simulink model "apf_pll"  (R2018a)
settings: Solver=ode1  StartTime=0  StopTime=40e-3  MaxStep=0.01  RelTol=0.1e-3
values from neighbouring files (symbols this model uses):
  R2 = 2    [mathematical_analysis.m]
undefined symbols (not defined in the file or in its folder): fs, pp
libraries: fl_lib x52, nesl_utility x17, powerlib x14, elec_lib x6, powerlib_extras x4, simulink x4, powerlib_meascontrol x1
settings Model: Creator=rodrigo  LastModifiedBy=LASAGNA
settings SolverCC: MaxConsecutiveZCs=10000  ShapePreserveControl=EnableAll  ZeroCrossControl=EnableAll
settings DataIOCC: SaveFormat=Array  SignalLoggingSaveFormat=ModelDataLogs  SaveOutput=off  SaveTime=off
settings OptimizationCC: BooleanDataType=off  ExpressionDepthLimit=2147483647  InitFltsAndDblsToZero=on  LifeSpan=inf
settings DebuggingCC: SaveWithParameterizedLinksMsg=none  UnderspecifiedInitializationDetection=Classic  MergeDetectMultiDrivingBlocksExec=none  SignalResolutionControl=TryResolveAllWithWarning  MultiTaskDSMMsg=warning  MultiTaskCondExecSysMsg=none  FcnCallInpInsideContextMsg=warning  StateNameClashWarn=warning  SFUnexpectedBacktrackingDiag=warning  SFNoUnconditionalDefaultTransitionDiag=warning  SFExecutionAtInitializationDiag=none
settings HardwareCC: ProdBitPerPointer=32  ProdBitPerSizeT=32  ProdBitPerPtrDiffT=32  ProdLargestAtomicFloat=None  ProdIntDivRoundTo=Undefined  ProdEndianess=Unspecified  ProdWordSize=32  ProdHWDeviceType=32-bit Generic  TargetBitPerPointer=64  TargetBitPerSizeT=64  TargetBitPerPtrDiffT=64  TargetLongLongMode=on  TargetIntDivRoundTo=Zero  TargetEndianess=LittleEndian  TargetWordSize=64  TargetHWDeviceType=MATLAB Host  ProdEqTarget=off
settings ModelReferenceCC: PropagateSignalLabelsOutOfModel=off
settings CodeAppCC: StateflowObjectComments=on
settings GRTTargetCC: TargetFcnLib=ansi_tfl_tmw.mat  TargetLangStandard=C89/C90 (ANSI)  CombineOutputUpdateFcns=off  GRTInterface=on
settings ConfigComp: CovMetricSettings=dw  CovHtmlReporting=on  CovSaveCumulativeToWorkspaceVar=on  CovSaveSingleToWorkspaceVar=on  CovExternalEMLEnable=off
settings SimscapeCC: SimscapeNormalizeSystem=off

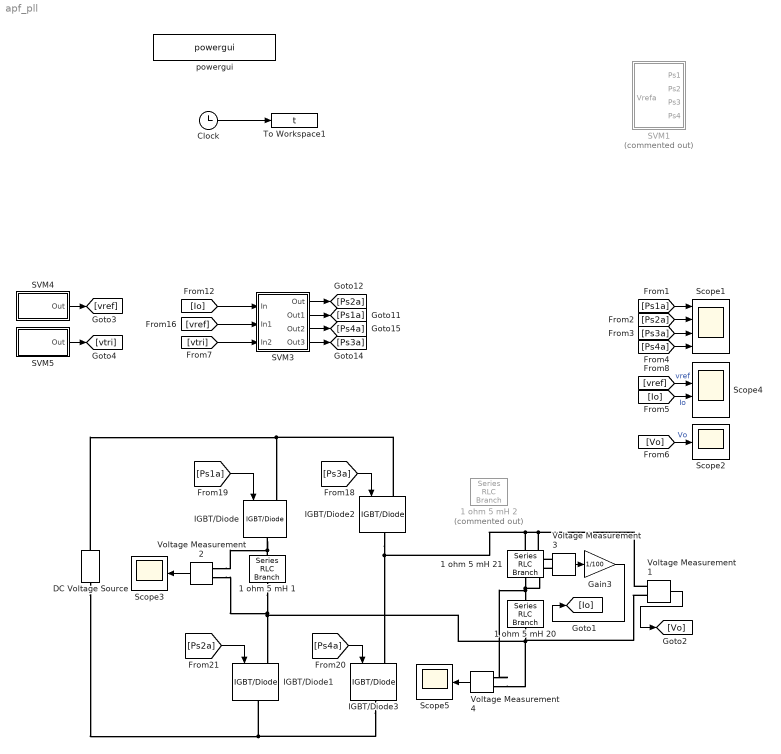
== system apf_pll ==
  1 ohm 5 mH 1 : powerlib/Elements/Series RLC Branch  LConnTagsString=__new0  RConnTagsString=__new0  BranchType=R  Resistance=1  Inductance=5e-03  SetiL0=off  InitialCurrent=0  Capacitance=0.001  Setx0=off  InitialVoltage=0  Measurements=None
  1 ohm 5 mH 2 : powerlib/Elements/Series RLC Branch  Commented=on  LConnTagsString=__new0  RConnTagsString=__new0  BranchType=R  Resistance=R2  Inductance=5e-03  SetiL0=off  InitialCurrent=0  Capacitance=0.001  Setx0=off  InitialVoltage=0  Measurements=None
  1 ohm 5 mH 20 : powerlib/Elements/Series RLC Branch  LConnTagsString=__new0  RConnTagsString=__new0  BranchType=L  Resistance=100  Inductance=0.256  SetiL0=off  InitialCurrent=10  Capacitance=60u  Setx0=off  InitialVoltage=0  Measurements=None
  1 ohm 5 mH 21 : powerlib/Elements/Series RLC Branch  LConnTagsString=__new0  RConnTagsString=__new0  BranchType=R  Resistance=100  Inductance=5e-03  SetiL0=off  InitialCurrent=0  Capacitance=0.001  Setx0=off  InitialVoltage=0  Measurements=None
  Clock : Clock
  DC Voltage Source : powerlib/Electrical Sources/DC Voltage Source  Amplitude=60  Measurements=None
  Gain3 : Gain  Gain=1/100
  IGBT/Diode{,1..3} (4 alike) : powerlib/Power Electronics/IGBT//Diode  Ron=1e-3  Rs=1e5  Cs=inf  Measurements=off
  SVM1 : Subsystem  Commented=on
  SVM3 : Subsystem
  SVM4 : Subsystem
  SVM5 : Subsystem
  Scope1 : Scope  NumInputPorts=4
  Scope2 : Scope
  Scope3 : Scope
  Scope4 : Scope  NumInputPorts=4
  Scope5 : Scope
  To Workspace1 : ToWorkspace  VariableName=t
      settings: MaxDataPoints=2000000
  Voltage Measurement{1..4} (4 alike) : powerlib/Measurements/Voltage Measurement  PhasorSimulation=off  OutputType=Complex  PSBequivalent=0
  powergui : powerlib/powergui  Priority=1  SimulationMode=Discrete  SampleTime=1/150e4  frequency=60  Iterations=50  frequencyindice=0  Pbase=100e6  ErrMax=1e-4  UnitsV=kV  UnitsW=MW  buscounter=0  FunctionMessages=off  echomessages=off  EnableUseOfTLC=off  CurrentSourceSwitches=off  DisableSnubberDevices=off  DisableRonSwitches=off  DisableVfSwitches=off  DisplayEquations=off  SolverType=Tustin/Backward Euler (TBE)  Interpol=off  ExternalGateDelay=off  methode=off  Ts=0  x0status=blocks  SPID=on  SwTol=0  HookPort=off  RestoreLinks=warning  ResistiveCurrentMeasurement=off  Frange=[0:2:500]  Ylog=off  Xlog=on  ShowGrid=off  save=off  variable=ZData  structure=ISA  ZoomFFT=off  StartTime=0.1  cycles=3  DisplayStyle=1  fundamental=60  FreqAxis=off  MaxFrequency=1000  frequencyindicesteady=1  RmsSteady=1  display=off
  wires:
  Clock/1 -> To Workspace1/1
  [Ps3a] -> IGBT/Diode2/1
  [Ps1a] -> IGBT/Diode/1
  [Ps4a] -> IGBT/Diode3/1
  [Ps2a] -> IGBT/Diode1/1
  [Ps1a] -> Scope1/1
  [Ps2a] -> Scope1/2
  [Ps3a] -> Scope1/3
  [Ps4a] -> Scope1/4
  Voltage Measurement3/1 -> Gain3/1
  Gain3/1 -> [Io]
  Voltage Measurement1/1 -> [Vo]
  SVM4/1(Out) -> [vref]
  [Vo] -> Scope2/1  "Vo"
  [vref] -> Scope4/2  "vref"
  [Io] -> Scope4/3  "Io"
  ? -> Scope4/1  "err"
  [Io] -> SVM3/1(In)
  ? -> Scope4/4  "IoxKh"
  [vref] -> SVM3/2(In1)
  SVM5/1(Out) -> [vtri]
  [vtri] -> SVM3/3(In2)
  SVM3/4(Out3) -> [Ps3a]
  SVM3/3(Out2) -> [Ps4a]
  SVM3/1(Out) -> [Ps2a]
  SVM3/2(Out1) -> [Ps1a]
  Voltage Measurement2/1 -> Scope3/1
  Voltage Measurement4/1 -> Scope5/1
  connections:
  Voltage Measurement1/LConn2 -- Voltage Measurement4/LConn2 -- 1 ohm 5 mH 20/LConn1 -- 1 ohm 5 mH 1/LConn1 -- Voltage Measurement2/LConn2 -- IGBT/Diode1/LConn1
  IGBT/Diode3/RConn1 -- IGBT/Diode1/RConn1 -- DC Voltage Source/LConn1
  IGBT/Diode2/LConn1 -- IGBT/Diode/LConn1 -- DC Voltage Source/RConn1
  1 ohm 5 mH 21/LConn1 -- 1 ohm 5 mH 20/RConn1 -- Voltage Measurement3/LConn2 -- Voltage Measurement4/LConn1
  1 ohm 5 mH 21/RConn1 -- Voltage Measurement1/LConn1 -- Voltage Measurement3/LConn1 -- IGBT/Diode2/RConn1 -- IGBT/Diode3/LConn1
  1 ohm 5 mH 1/RConn1 -- Voltage Measurement2/LConn1 -- IGBT/Diode/RConn1

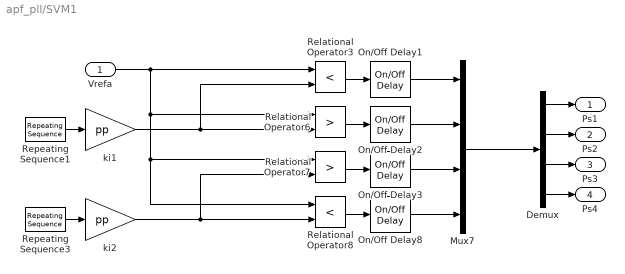
== system apf_pll/SVM1 ==
  Vrefa : Inport
  Demux : Demux
  Mux7 : Mux
  On/Off Delay{1..3,8} (4 alike) : powerlib_extras/Control  Blocks/On//Off Delay  type_delay=On delay  delay=tm  ic=0
  Relational Operator3 : RelationalOperator  Operator=<  OutDataTypeStr=boolean  RndMeth=Nearest
  Relational Operator6 : RelationalOperator  Operator=>  OutDataTypeStr=boolean  RndMeth=Nearest
  Relational Operator7 : RelationalOperator  Operator=>  OutDataTypeStr=boolean  RndMeth=Nearest
  Relational Operator8 : RelationalOperator  Operator=<  OutDataTypeStr=boolean  RndMeth=Nearest
  Repeating Sequence1 : simulink/Sources/Repeating Sequence  rep_seq_t=[0 1/(2*fs) 1/fs]  rep_seq_y=[0 1 0]
  Repeating Sequence3 : simulink/Sources/Repeating Sequence  rep_seq_t=[0 1/(2*fs) 1/fs]  rep_seq_y=[1 0 1]
  ki1 : Gain  Gain=pp  SaturateOnIntegerOverflow=on  OutDataTypeStr=Inherit: Same as input  ParamDataTypeStr=Inherit: Same as input
  ki2 : Gain  Gain=pp  SaturateOnIntegerOverflow=on  OutDataTypeStr=Inherit: Same as input  ParamDataTypeStr=Inherit: Same as input
  Ps1 : Outport
  Ps2 : Outport  Port=2
  Ps3 : Outport  Port=3
  Ps4 : Outport  Port=4
  wires:
  Vrefa/1 -> Relational Operator3/1, Relational Operator7/1, Relational Operator8/1, Relational Operator6/1
  Repeating Sequence1/1 -> ki1/1
  ki1/1 -> Relational Operator3/2, Relational Operator6/2
  ki2/1 -> Relational Operator8/2, Relational Operator7/2
  Repeating Sequence3/1 -> ki2/1
  Relational Operator3/1 -> On/Off Delay1/1
  Relational Operator6/1 -> On/Off Delay2/1
  Relational Operator7/1 -> On/Off Delay3/1
  Relational Operator8/1 -> On/Off Delay8/1
  On/Off Delay2/1 -> Mux7/2
  On/Off Delay1/1 -> Mux7/1
  On/Off Delay3/1 -> Mux7/3
  On/Off Delay8/1 -> Mux7/4
  Demux/1 -> Ps1/1
  Demux/2 -> Ps2/1
  Demux/3 -> Ps3/1
  Demux/4 -> Ps4/1
  Mux7/1 -> Demux/1

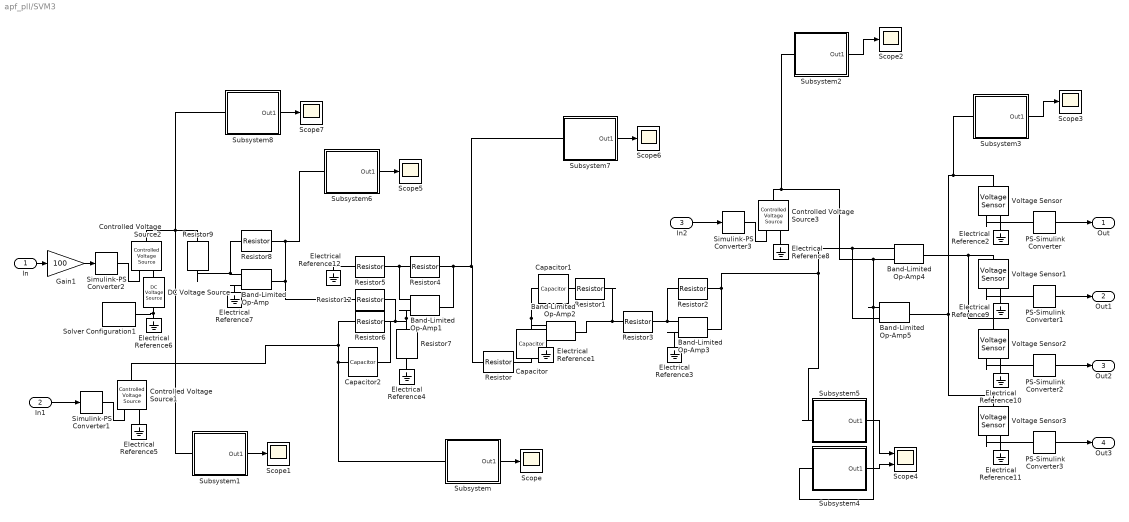
== system apf_pll/SVM3 ==
  In : Inport
  In1 : Inport  Port=2
  In2 : Inport  Port=3
  Band-Limited Op-Amp{,1..3} (4 alike) : elec_lib/Integrated Circuits/Band-Limited Op-Amp  A=25000  Rin=1e12 Ohm  Rout=50 Ohm  Vmin=-15 V  Vmax=15 V  Vdotmax=1e5 V/s  f=3 GHz  V0=0 V
      settings: SourceProductName=Simscape Electronics  SourceProductBaseCode=SN
  Band-Limited Op-Amp4 : elec_lib/Integrated Circuits/Band-Limited Op-Amp  A=25000  Rin=1e12 Ohm  Rout=50 Ohm  Vmin=0 V  Vmax=5 V  Vdotmax=1e5 V/s  f=3 GHz  V0=0 V
      settings: SourceProductName=Simscape Electronics  SourceProductBaseCode=SN
  Band-Limited Op-Amp5 : elec_lib/Integrated Circuits/Band-Limited Op-Amp  A=25000  Rin=1e12 Ohm  Rout=50 Ohm  Vmin=0 V  Vmax=5 V  Vdotmax=1e5 V/s  f=3 GHz  V0=0 V
      settings: SourceProductName=Simscape Electronics  SourceProductBaseCode=SN
  Capacitor : fl_lib/Electrical/Electrical Elements/Capacitor  c=100 nF  r=1e-6 Ohm  g=1e-9 1/Ohm  i_specify=off  i_priority=None  i=0 A  i_nominal_specify=off  i_nominal_unit=A  i_nominal_value=1  v_specify=off  v_priority=None  v=0 V  v_nominal_specify=off  v_nominal_unit=V  v_nominal_value=1  vc_specify=off  vc_priority=High  vc=0 V  vc_nominal_specify=off  vc_nominal_unit=V  vc_nominal_value=1
  Capacitor1 : fl_lib/Electrical/Electrical Elements/Capacitor  c=100 nF  r=1e-6 Ohm  g=1e-9 1/Ohm  i_specify=off  i_priority=None  i=0 A  i_nominal_specify=off  i_nominal_unit=A  i_nominal_value=1  v_specify=off  v_priority=None  v=0 V  v_nominal_specify=off  v_nominal_unit=V  v_nominal_value=1  vc_specify=off  vc_priority=High  vc=0 V  vc_nominal_specify=off  vc_nominal_unit=V  vc_nominal_value=1
  Capacitor2 : fl_lib/Electrical/Electrical Elements/Capacitor  c=100 nF  r=1e-6 Ohm  g=1e-9 1/Ohm  i_specify=off  i_priority=None  i=0 A  i_nominal_specify=off  i_nominal_unit=A  i_nominal_value=1  v_specify=off  v_priority=None  v=0 V  v_nominal_specify=off  v_nominal_unit=V  v_nominal_value=1  vc_specify=off  vc_priority=High  vc=0 V  vc_nominal_specify=off  vc_nominal_unit=V  vc_nominal_value=1
  Controlled Voltage Source1 : fl_lib/Electrical/Electrical Sources/Controlled Voltage Source
  Controlled Voltage Source2 : fl_lib/Electrical/Electrical Sources/Controlled Voltage Source
  Controlled Voltage Source3 : fl_lib/Electrical/Electrical Sources/Controlled Voltage Source
  DC Voltage Source : fl_lib/Electrical/Electrical Sources/DC Voltage Source  v0=0 V
  Electrical Reference{1..12} (12 alike) : fl_lib/Electrical/Electrical Elements/Electrical Reference
  Gain1 : Gain  Gain=100
  PS-Simulink Converter{,1..3} (4 alike) : nesl_utility/PS-Simulink Converter  PhysicalDomain=network_engine_domain  SubClassName=ps_output  LeftPortType=input  RightPortType=output  PseudoPeriodic=off  Frequencies=[]  Unit=1  AffineConversion=off
  Resistor : fl_lib/Electrical/Electrical Elements/Resistor  R=54.9 kOhm  i_specify=off  i_priority=None  i=0 A  i_nominal_specify=off  i_nominal_unit=A  i_nominal_value=1  v_specify=off  v_priority=None  v=0 V  v_nominal_specify=off  v_nominal_unit=V  v_nominal_value=1
  Resistor1 : fl_lib/Electrical/Electrical Elements/Resistor  R=12.8 kOhm  i_specify=off  i_priority=None  i=0 A  i_nominal_specify=off  i_nominal_unit=A  i_nominal_value=1  v_specify=off  v_priority=None  v=0 V  v_nominal_specify=off  v_nominal_unit=V  v_nominal_value=1
  Resistor{4..7,12} (5 alike) : fl_lib/Electrical/Electrical Elements/Resistor  R=20 kOhm  i_specify=off  i_priority=None  i=0 A  i_nominal_specify=off  i_nominal_unit=A  i_nominal_value=1  v_specify=off  v_priority=None  v=0 V  v_nominal_specify=off  v_nominal_unit=V  v_nominal_value=1
  Resistor2 : fl_lib/Electrical/Electrical Elements/Resistor  R=10 kOhm  i_specify=off  i_priority=None  i=0 A  i_nominal_specify=off  i_nominal_unit=A  i_nominal_value=1  v_specify=off  v_priority=None  v=0 V  v_nominal_specify=off  v_nominal_unit=V  v_nominal_value=1
  Resistor3 : fl_lib/Electrical/Electrical Elements/Resistor  R=1 kOhm  i_specify=off  i_priority=None  i=0 A  i_nominal_specify=off  i_nominal_unit=A  i_nominal_value=1  v_specify=off  v_priority=None  v=0 V  v_nominal_specify=off  v_nominal_unit=V  v_nominal_value=1
  Resistor8 : fl_lib/Electrical/Electrical Elements/Resistor  R=10 kOhm  i_specify=off  i_priority=None  i=0 A  i_nominal_specify=off  i_nominal_unit=A  i_nominal_value=1  v_specify=off  v_priority=None  v=0 V  v_nominal_specify=off  v_nominal_unit=V  v_nominal_value=1
  Resistor9 : fl_lib/Electrical/Electrical Elements/Resistor  R=100 kOhm  i_specify=off  i_priority=None  i=0 A  i_nominal_specify=off  i_nominal_unit=A  i_nominal_value=1  v_specify=off  v_priority=None  v=0 V  v_nominal_specify=off  v_nominal_unit=V  v_nominal_value=1
  Scope{,1..3,5..7} (7 alike) : Scope
  Scope4 : Scope  NumInputPorts=2
  Simulink-PS Converter1 : nesl_utility/Simulink-PS Converter  PhysicalDomain=network_engine_domain  SubClassName=ps_input  LeftPortType=input  RightPortType=output  PseudoPeriodic=off  Frequencies=[]  NoiseDistribution=none  NoiseParameters=[]  Unit=1  AffineConversion=off  FilteringAndDerivatives=provide  SimscapeFilterOrder=1  InputFilterTimeConstant=0.001  UdotUserProvided=0
  Simulink-PS Converter2 : nesl_utility/Simulink-PS Converter  PhysicalDomain=network_engine_domain  SubClassName=ps_input  LeftPortType=input  RightPortType=output  PseudoPeriodic=off  Frequencies=[]  NoiseDistribution=none  NoiseParameters=[]  Unit=1  AffineConversion=off  FilteringAndDerivatives=provide  SimscapeFilterOrder=1  InputFilterTimeConstant=0.001  UdotUserProvided=0
  Simulink-PS Converter3 : nesl_utility/Simulink-PS Converter  PhysicalDomain=network_engine_domain  SubClassName=ps_input  LeftPortType=input  RightPortType=output  PseudoPeriodic=off  Frequencies=[]  NoiseDistribution=none  NoiseParameters=[]  Unit=1  AffineConversion=off  FilteringAndDerivatives=provide  SimscapeFilterOrder=1  InputFilterTimeConstant=0.001  UdotUserProvided=0
  Solver Configuration1 : nesl_utility/Solver Configuration  PhysicalDomain=network_engine_domain  SubClassName=solver  LeftPortType=input  RightPortType=generic  Tones=[]  Harmonics=[]  SimulateNoise=off  Profile=off  UseLocalSampling=off  EnableSwitchedLinearOptims=on  FrequencyDomain=off  UseCCode=off  RelTol=0.001  AbsTol=1e-06  MinStep=1e-09  ToWorkspace=off  RevertToSquareIcSolve=off  NumHomotopyIterations=100  PhasorMode=off  PhasorModeNumHarmonics=1  DoDC=off  ResidualTolerance=1e-09  UseLocalSolver=off  LocalSolverChoice=NE_BACKWARD_EULER_ADVANCER  LocalSolverSampleTime=0.001  DoFixedCost=off  MaxNonlinIter=3  MaxModeIter=2  LinearAlgebra=Sparse  EquationFormulation=NE_TIME_EF  DelaysMemoryBudget=1024  AutomaticFiltering=on  FilteringTimeConstant=0.001
  Subsystem : Subsystem
  Subsystem1 : Subsystem
  Subsystem2 : Subsystem
  Subsystem3 : Subsystem
  Subsystem4 : Subsystem
  Subsystem5 : Subsystem
  Subsystem6 : Subsystem
  Subsystem7 : Subsystem
  Subsystem8 : Subsystem
  Voltage Sensor{,1..3} (4 alike) : fl_lib/Electrical/Electrical Sensors/Voltage Sensor
  Out : Outport
  Out1 : Outport  Port=2
  Out2 : Outport  Port=3
  Out3 : Outport  Port=4
  wires:
  PS-Simulink Converter/1 -> Out/1
  In1/1 -> Simulink-PS Converter1/1
  Gain1/1 -> Simulink-PS Converter2/1
  In/1 -> Gain1/1
  Subsystem/1(Out1) -> Scope/1
  Subsystem1/1(Out1) -> Scope1/1
  In2/1 -> Simulink-PS Converter3/1
  PS-Simulink Converter1/1 -> Out1/1
  PS-Simulink Converter2/1 -> Out2/1
  PS-Simulink Converter3/1 -> Out3/1
  Subsystem2/1(Out1) -> Scope2/1
  Subsystem3/1(Out1) -> Scope3/1
  Subsystem4/1(Out1) -> Scope4/2
  Subsystem5/1(Out1) -> Scope4/1
  Subsystem6/1(Out1) -> Scope5/1
  Subsystem7/1(Out1) -> Scope6/1
  Subsystem8/1(Out1) -> Scope7/1
  connections:
  Resistor4/RConn1 -- Band-Limited Op-Amp1/RConn1 -- Subsystem7/LConn1 -- Resistor/LConn1
  Resistor2/LConn1 -- Band-Limited Op-Amp3/LConn2 -- Resistor3/RConn1
  Voltage Sensor/RConn1 -- PS-Simulink Converter/LConn1
  Voltage Sensor/RConn2 -- Electrical Reference2/LConn1
  Capacitor/LConn1 -- Band-Limited Op-Amp2/LConn2 -- Capacitor1/RConn1
  Band-Limited Op-Amp2/LConn1 -- Electrical Reference1/LConn1
  Resistor1/RConn1 -- Band-Limited Op-Amp2/RConn1 -- Resistor3/LConn1
  Controlled Voltage Source3/LConn1 -- Band-Limited Op-Amp4/LConn1 -- Band-Limited Op-Amp5/LConn2 -- Subsystem4/LConn1 -- Subsystem2/LConn1
  Band-Limited Op-Amp3/LConn1 -- Electrical Reference3/LConn1
  Resistor5/RConn1 -- Band-Limited Op-Amp1/LConn2 -- Resistor4/LConn1
  Resistor7/RConn1 -- Electrical Reference4/LConn1
  Resistor7/LConn1 -- Band-Limited Op-Amp1/LConn1 -- Resistor12/RConn1 -- Capacitor2/LConn1 -- Resistor6/RConn1
  Controlled Voltage Source1/RConn1 -- Simulink-PS Converter1/RConn1
  Electrical Reference5/LConn1 -- Controlled Voltage Source1/RConn2
  Resistor6/LConn1 -- Capacitor2/RConn1 -- Subsystem/LConn1 -- Controlled Voltage Source1/LConn1
  Controlled Voltage Source2/RConn1 -- Simulink-PS Converter2/RConn1
  DC Voltage Source/LConn1 -- Controlled Voltage Source2/RConn2
  Electrical Reference6/LConn1 -- Solver Configuration1/RConn1 -- DC Voltage Source/RConn1
  Resistor8/LConn1 -- Band-Limited Op-Amp/LConn2 -- Resistor9/RConn1
  Resistor8/RConn1 -- Subsystem6/LConn1 -- Band-Limited Op-Amp/RConn1 -- Resistor12/LConn1
  Controlled Voltage Source2/LConn1 -- Subsystem8/LConn1 -- Resistor9/LConn1 -- Subsystem1/LConn1
  Electrical Reference8/LConn1 -- Controlled Voltage Source3/RConn2
  Controlled Voltage Source3/RConn1 -- Simulink-PS Converter3/RConn1
  Voltage Sensor1/RConn1 -- PS-Simulink Converter1/LConn1
  Voltage Sensor1/RConn2 -- Electrical Reference9/LConn1
  Voltage Sensor2/RConn1 -- PS-Simulink Converter2/LConn1
  Voltage Sensor2/RConn2 -- Electrical Reference10/LConn1
  Voltage Sensor3/RConn1 -- PS-Simulink Converter3/LConn1
  Voltage Sensor3/RConn2 -- Electrical Reference11/LConn1
  Voltage Sensor3/LConn1 -- Band-Limited Op-Amp5/RConn1 -- Subsystem3/LConn1 -- Voltage Sensor/LConn1
  Voltage Sensor2/LConn1 -- Band-Limited Op-Amp4/RConn1 -- Voltage Sensor1/LConn1
  Subsystem5/LConn1 -- Band-Limited Op-Amp5/LConn1 -- Band-Limited Op-Amp4/LConn2 -- Band-Limited Op-Amp3/RConn1 -- Resistor2/RConn1
  Capacitor1/LConn1 -- Resistor1/LConn1
  Resistor/RConn1 -- Capacitor/RConn1
  Band-Limited Op-Amp/LConn1 -- Electrical Reference7/LConn1
  Resistor5/LConn1 -- Electrical Reference12/LConn1

== system apf_pll/SVM4 ==
  Add : Sum
  Band-Limited White Noise : simulink/Sources/Band-Limited White Noise  Cov=[1e-9]  Ts=1e-6  seed=[23341]
  Sine Wave : Sin  Frequency=377  SampleTime=0
  Out : Outport
  wires:
  Band-Limited White Noise/1 -> Add/2
  Add/1 -> Out/1
  Sine Wave/1 -> Add/1

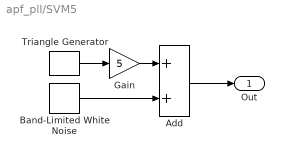
== system apf_pll/SVM5 ==
  Add : Sum
  Band-Limited White Noise : simulink/Sources/Band-Limited White Noise  Cov=[1e-6]  Ts=1e-6  seed=[23341]
  Gain : Gain  Gain=5
  Triangle Generator : powerlib_meascontrol/Pulse & Signal Generators/Triangle Generator  Freq=1000  Phase=90  Ts=0
  Out : Outport
  wires:
  Band-Limited White Noise/1 -> Add/2
  Add/1 -> Out/1
  Gain/1 -> Add/1
  Triangle Generator/1 -> Gain/1

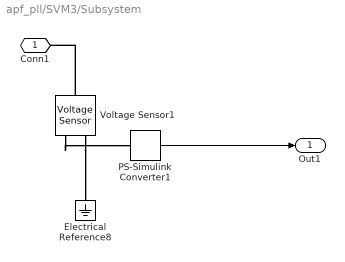
== system apf_pll/SVM3/Subsystem ==
  Electrical Reference8 : fl_lib/Electrical/Electrical Elements/Electrical Reference
  PS-Simulink Converter1 : nesl_utility/PS-Simulink Converter  PhysicalDomain=network_engine_domain  SubClassName=ps_output  LeftPortType=input  RightPortType=output  PseudoPeriodic=off  Frequencies=[]  Unit=1  AffineConversion=off
  Voltage Sensor1 : fl_lib/Electrical/Electrical Sensors/Voltage Sensor
  Conn1 : PMIOPort  Side=Left
  Out1 : Outport
  wires:
  PS-Simulink Converter1/1 -> Out1/1
  connections:
  Voltage Sensor1/RConn1 -- PS-Simulink Converter1/LConn1
  Voltage Sensor1/RConn2 -- Electrical Reference8/LConn1
  Voltage Sensor1/LConn1 -- Conn1/RConn1

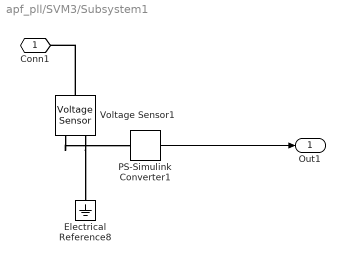
== system apf_pll/SVM3/Subsystem1 ==
  Electrical Reference8 : fl_lib/Electrical/Electrical Elements/Electrical Reference
  PS-Simulink Converter1 : nesl_utility/PS-Simulink Converter  PhysicalDomain=network_engine_domain  SubClassName=ps_output  LeftPortType=input  RightPortType=output  PseudoPeriodic=off  Frequencies=[]  Unit=1  AffineConversion=off
  Voltage Sensor1 : fl_lib/Electrical/Electrical Sensors/Voltage Sensor
  Conn1 : PMIOPort  Side=Left
  Out1 : Outport
  wires:
  PS-Simulink Converter1/1 -> Out1/1
  connections:
  Voltage Sensor1/RConn1 -- PS-Simulink Converter1/LConn1
  Voltage Sensor1/RConn2 -- Electrical Reference8/LConn1
  Voltage Sensor1/LConn1 -- Conn1/RConn1

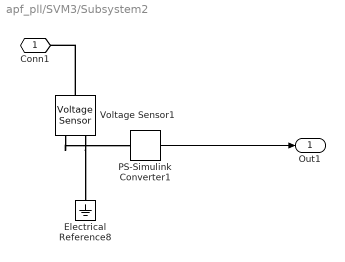
== system apf_pll/SVM3/Subsystem2 ==
  Electrical Reference8 : fl_lib/Electrical/Electrical Elements/Electrical Reference
  PS-Simulink Converter1 : nesl_utility/PS-Simulink Converter  PhysicalDomain=network_engine_domain  SubClassName=ps_output  LeftPortType=input  RightPortType=output  PseudoPeriodic=off  Frequencies=[]  Unit=1  AffineConversion=off
  Voltage Sensor1 : fl_lib/Electrical/Electrical Sensors/Voltage Sensor
  Conn1 : PMIOPort  Side=Left
  Out1 : Outport
  wires:
  PS-Simulink Converter1/1 -> Out1/1
  connections:
  Voltage Sensor1/RConn1 -- PS-Simulink Converter1/LConn1
  Voltage Sensor1/RConn2 -- Electrical Reference8/LConn1
  Voltage Sensor1/LConn1 -- Conn1/RConn1

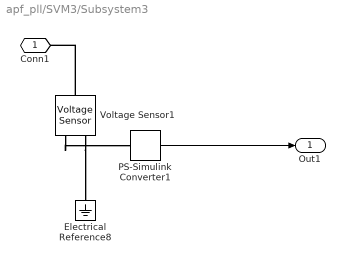
== system apf_pll/SVM3/Subsystem3 ==
  Electrical Reference8 : fl_lib/Electrical/Electrical Elements/Electrical Reference
  PS-Simulink Converter1 : nesl_utility/PS-Simulink Converter  PhysicalDomain=network_engine_domain  SubClassName=ps_output  LeftPortType=input  RightPortType=output  PseudoPeriodic=off  Frequencies=[]  Unit=1  AffineConversion=off
  Voltage Sensor1 : fl_lib/Electrical/Electrical Sensors/Voltage Sensor
  Conn1 : PMIOPort  Side=Left
  Out1 : Outport
  wires:
  PS-Simulink Converter1/1 -> Out1/1
  connections:
  Voltage Sensor1/RConn1 -- PS-Simulink Converter1/LConn1
  Voltage Sensor1/RConn2 -- Electrical Reference8/LConn1
  Voltage Sensor1/LConn1 -- Conn1/RConn1

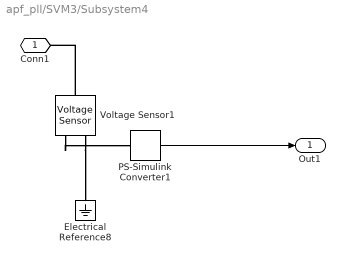
== system apf_pll/SVM3/Subsystem4 ==
  Electrical Reference8 : fl_lib/Electrical/Electrical Elements/Electrical Reference
  PS-Simulink Converter1 : nesl_utility/PS-Simulink Converter  PhysicalDomain=network_engine_domain  SubClassName=ps_output  LeftPortType=input  RightPortType=output  PseudoPeriodic=off  Frequencies=[]  Unit=1  AffineConversion=off
  Voltage Sensor1 : fl_lib/Electrical/Electrical Sensors/Voltage Sensor
  Conn1 : PMIOPort  Side=Left
  Out1 : Outport
  wires:
  PS-Simulink Converter1/1 -> Out1/1
  connections:
  Voltage Sensor1/RConn1 -- PS-Simulink Converter1/LConn1
  Voltage Sensor1/RConn2 -- Electrical Reference8/LConn1
  Voltage Sensor1/LConn1 -- Conn1/RConn1

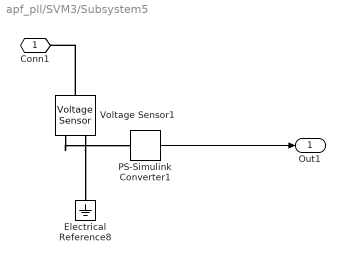
== system apf_pll/SVM3/Subsystem5 ==
  Electrical Reference8 : fl_lib/Electrical/Electrical Elements/Electrical Reference
  PS-Simulink Converter1 : nesl_utility/PS-Simulink Converter  PhysicalDomain=network_engine_domain  SubClassName=ps_output  LeftPortType=input  RightPortType=output  PseudoPeriodic=off  Frequencies=[]  Unit=1  AffineConversion=off
  Voltage Sensor1 : fl_lib/Electrical/Electrical Sensors/Voltage Sensor
  Conn1 : PMIOPort  Side=Left
  Out1 : Outport
  wires:
  PS-Simulink Converter1/1 -> Out1/1
  connections:
  Voltage Sensor1/RConn1 -- PS-Simulink Converter1/LConn1
  Voltage Sensor1/RConn2 -- Electrical Reference8/LConn1
  Voltage Sensor1/LConn1 -- Conn1/RConn1

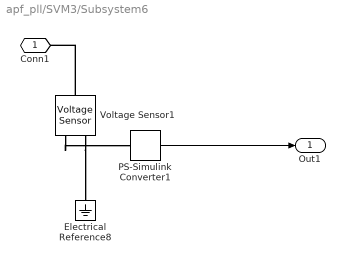
== system apf_pll/SVM3/Subsystem6 ==
  Electrical Reference8 : fl_lib/Electrical/Electrical Elements/Electrical Reference
  PS-Simulink Converter1 : nesl_utility/PS-Simulink Converter  PhysicalDomain=network_engine_domain  SubClassName=ps_output  LeftPortType=input  RightPortType=output  PseudoPeriodic=off  Frequencies=[]  Unit=1  AffineConversion=off
  Voltage Sensor1 : fl_lib/Electrical/Electrical Sensors/Voltage Sensor
  Conn1 : PMIOPort  Side=Left
  Out1 : Outport
  wires:
  PS-Simulink Converter1/1 -> Out1/1
  connections:
  Voltage Sensor1/RConn1 -- PS-Simulink Converter1/LConn1
  Voltage Sensor1/RConn2 -- Electrical Reference8/LConn1
  Voltage Sensor1/LConn1 -- Conn1/RConn1

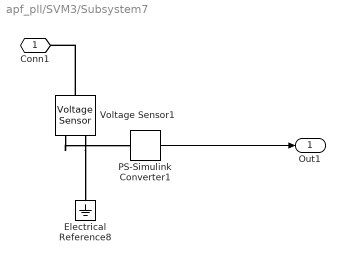
== system apf_pll/SVM3/Subsystem7 ==
  Electrical Reference8 : fl_lib/Electrical/Electrical Elements/Electrical Reference
  PS-Simulink Converter1 : nesl_utility/PS-Simulink Converter  PhysicalDomain=network_engine_domain  SubClassName=ps_output  LeftPortType=input  RightPortType=output  PseudoPeriodic=off  Frequencies=[]  Unit=1  AffineConversion=off
  Voltage Sensor1 : fl_lib/Electrical/Electrical Sensors/Voltage Sensor
  Conn1 : PMIOPort  Side=Left
  Out1 : Outport
  wires:
  PS-Simulink Converter1/1 -> Out1/1
  connections:
  Voltage Sensor1/RConn1 -- PS-Simulink Converter1/LConn1
  Voltage Sensor1/RConn2 -- Electrical Reference8/LConn1
  Voltage Sensor1/LConn1 -- Conn1/RConn1

== system apf_pll/SVM3/Subsystem8 ==
  Electrical Reference8 : fl_lib/Electrical/Electrical Elements/Electrical Reference
  PS-Simulink Converter1 : nesl_utility/PS-Simulink Converter  PhysicalDomain=network_engine_domain  SubClassName=ps_output  LeftPortType=input  RightPortType=output  PseudoPeriodic=off  Frequencies=[]  Unit=1  AffineConversion=off
  Voltage Sensor1 : fl_lib/Electrical/Electrical Sensors/Voltage Sensor
  Conn1 : PMIOPort  Side=Left
  Out1 : Outport
  wires:
  PS-Simulink Converter1/1 -> Out1/1
  connections:
  Voltage Sensor1/RConn1 -- PS-Simulink Converter1/LConn1
  Voltage Sensor1/RConn2 -- Electrical Reference8/LConn1
  Voltage Sensor1/LConn1 -- Conn1/RConn1
